simulink model "estimate_lane_center"  (R2019b)
settings: Solver=VariableStepAuto  StartTime=0.0  StopTime=10.0  RelTol=1e-3
undefined symbols (not defined in the file): PredictionHorizon, Ts
settings Model: Creator=senoa95  LastModifiedBy=senoa95

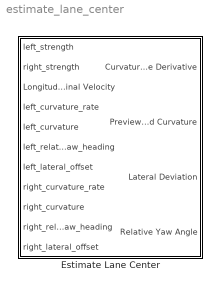
== system estimate_lane_center ==
  Estimate Lane Center : Subsystem  TreatAsAtomicUnit=on  VariantControl=v2
      settings: RTWFileNameOpts=Use function name

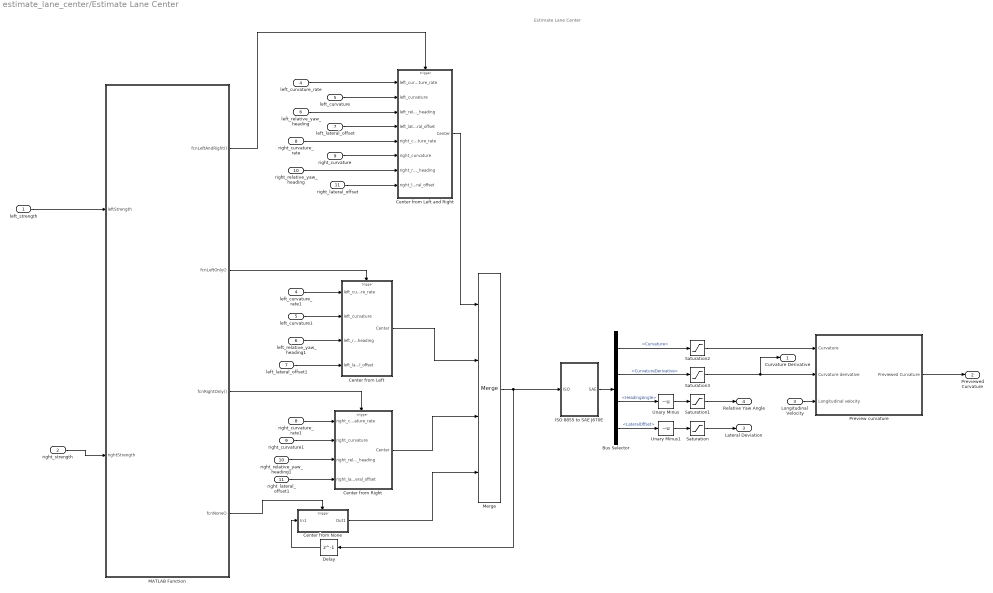
== system estimate_lane_center/Estimate Lane Center ==
  note: Estimate Lane Center
  left_strength : Inport
  right_strength : Inport  Port=2
  Longitudinal Velocity : Inport  Port=3
  left_curvature_rate : Inport  Port=4
  left_curvature : Inport  Port=5
  left_relative_yaw_heading : Inport  Port=6
  left_lateral_offset : Inport  Port=7
  right_curvature_rate : Inport  Port=8
  right_curvature : Inport  Port=9
  right_relative_yaw_heading : Inport  Port=10
  right_lateral_offset : Inport  Port=11
  Bus Selector : BusSelector  OutputSignals=Curvature,CurvatureDerivative,HeadingAngle,LateralOffset
  Center from Left : Subsystem  TreatAsAtomicUnit=on
  Center from Left and Right : Subsystem  TreatAsAtomicUnit=on
  Center from None : Subsystem  TreatAsAtomicUnit=on
  Center from Right : Subsystem  TreatAsAtomicUnit=on
  Delay : Delay  DelayLength=1
  ISO 8855 to SAE J670E : Subsystem
  MATLAB Function : MATLAB Function  TreatAsAtomicUnit=on
  Merge : Merge  Inputs=4
  Preview curvature : Subsystem
  Saturation : Saturate
  Saturation1 : Saturate  UpperLimit=0.6  LowerLimit=-0.6
  Saturation2 : Saturate  UpperLimit=0.15  LowerLimit=-0.15
  Saturation3 : Saturate  UpperLimit=0.06  LowerLimit=-0.06
  Unary Minus : UnaryMinus
  Unary Minus1 : UnaryMinus
  left_curvature1 : InportShadow  Port=5
  left_curvature_rate1 : InportShadow  Port=4
  left_lateral_offset1 : InportShadow  Port=7
  left_relative_yaw_heading1 : InportShadow  Port=6
  right_curvature1 : InportShadow  Port=9
  right_curvature_rate1 : InportShadow  Port=8
  right_lateral_offset1 : InportShadow  Port=11
  right_relative_yaw_heading1 : InportShadow  Port=10
  Curvature Derivative : Outport
  Previewed Curvature : Outport  Port=2  VectorParamsAs1DForOutWhenUnconnected=off
  Lateral Deviation : Outport  Port=3  VectorParamsAs1DForOutWhenUnconnected=off
  Relative Yaw Angle : Outport  Port=4  VectorParamsAs1DForOutWhenUnconnected=off
  wires:
  Center from Right/1(Center) -> Merge/3
  MATLAB Function/2(fcnLeftOnly()) -> Center from Left/Trigger
  Center from None/1(Out1) -> Merge/4
  MATLAB Function/1(fcnLeftAndRight()) -> Center from Left and Right/Trigger
  Delay/1 -> Center from None/1(In1)
  Center from Left and Right/1(Center) -> Merge/1
  MATLAB Function/3(fcnRightOnly()) -> Center from Right/Trigger
  MATLAB Function/4(fcnNone()) -> Center from None/Trigger
  Center from Left/1(Center) -> Merge/2
  Merge/1 -> ISO 8855 to SAE J670E/1(ISO), Delay/1
  Saturation3/1 -> Curvature Derivative/1, Preview curvature/2(Curvature derivative)
  Saturation2/1 -> Preview curvature/1(Curvature)
  Saturation1/1 -> Relative Yaw Angle/1
  Saturation/1 -> Lateral Deviation/1
  Unary Minus/1 -> Saturation1/1
  Preview curvature/1(Previewed Curvature) -> Previewed Curvature/1
  Longitudinal Velocity/1 -> Preview curvature/3(Longitudinal velocity)
  Bus Selector/2 -> Saturation3/1  "<CurvatureDerivative>"
  Bus Selector/1 -> Saturation2/1  "<Curvature>"
  Unary Minus1/1 -> Saturation/1
  Bus Selector/4 -> Unary Minus1/1  "<LateralOffset>"
  Bus Selector/3 -> Unary Minus/1  "<HeadingAngle>"
  ISO 8855 to SAE J670E/1(SAE) -> Bus Selector/1
  left_strength/1 -> MATLAB Function/1(leftStrength)
  right_strength/1 -> MATLAB Function/2(rightStrength)
  left_curvature_rate/1 -> Center from Left and Right/1(left_curvature_rate)
  right_relative_yaw_heading/1 -> Center from Left and Right/7(right_relative_yaw_heading)
  right_lateral_offset/1 -> Center from Left and Right/8(right_lateral_offset)
  left_lateral_offset/1 -> Center from Left and Right/4(left_lateral_offset)
  left_curvature/1 -> Center from Left and Right/2(left_curvature)
  left_relative_yaw_heading/1 -> Center from Left and Right/3(left_relative_yaw_heading)
  right_curvature_rate/1 -> Center from Left and Right/5(right_curvature_rate)
  right_curvature/1 -> Center from Left and Right/6(right_curvature)
  left_curvature_rate1/1 -> Center from Left/1(left_curvature_rate)
  left_curvature1/1 -> Center from Left/2(left_curvature)
  left_relative_yaw_heading1/1 -> Center from Left/3(left_relative_yaw_heading)
  left_lateral_offset1/1 -> Center from Left/4(left_lateral_offset)
  right_curvature_rate1/1 -> Center from Right/1(right_curvature_rate)
  right_curvature1/1 -> Center from Right/2(right_curvature)
  right_relative_yaw_heading1/1 -> Center from Right/3(right_relative_yaw_heading)
  right_lateral_offset1/1 -> Center from Right/4(right_lateral_offset)

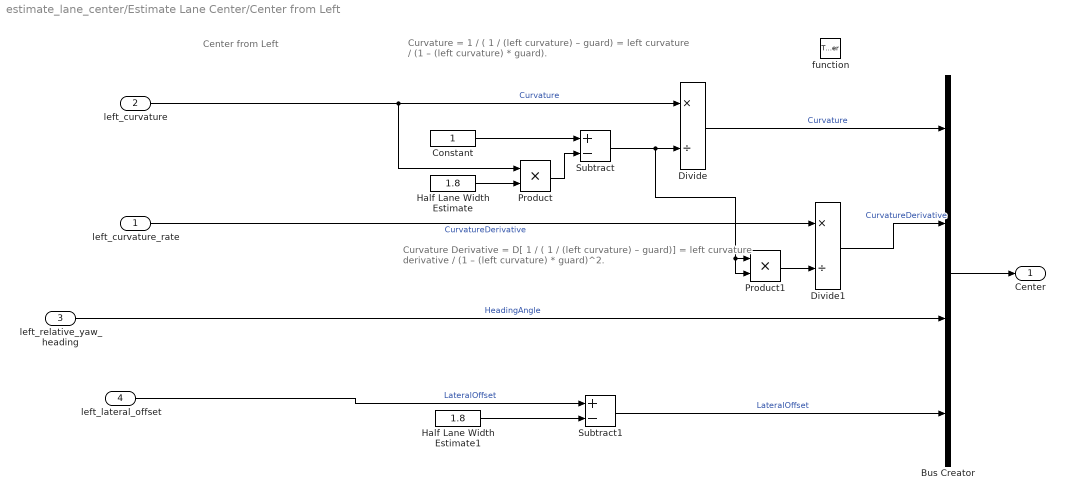
== system estimate_lane_center/Estimate Lane Center/Center from Left ==
  note: Curvature Derivative
      | = D[ 1 / ( 1 / (left curvature) – guard)]
      | = left curvature derivative / (1 – (left curvature) * guard)^2.
  note: Center from Left
  note: Curvature
      | = 1 / ( 1 / (left curvature) – guard)
      | = left curvature / (1 – (left curvature) * guard).
  left_curvature_rate : Inport
  left_curvature : Inport  Port=2
  left_relative_yaw_heading : Inport  Port=3
  left_lateral_offset : Inport  Port=4
  function : TriggerPort  TriggerType=function-call  VariantControl=Variant
  Bus Creator : BusCreator  Inputs=4
  Constant : Constant  OutDataTypeStr=Inherit: Inherit via back propagation
  Divide : Product  Inputs=*/
  Divide1 : Product  Inputs=*/
  Half Lane Width Estimate : Constant  Value=1.8  OutDataTypeStr=Inherit: Inherit via back propagation
  Half Lane Width Estimate1 : Constant  Value=1.8  OutDataTypeStr=Inherit: Inherit via back propagation
  Product : Product
  Product1 : Product
  Subtract : Sum  Inputs=+-
  Subtract1 : Sum  Inputs=+-
  Center : Outport  VectorParamsAs1DForOutWhenUnconnected=off
  wires:
  Product/1 -> Subtract/2
  Half Lane Width Estimate1/1 -> Subtract1/2
  left_lateral_offset/1 -> Subtract1/1  "LateralOffset"
  Product1/1 -> Divide1/2
  left_curvature_rate/1 -> Divide1/1  "CurvatureDerivative"
  Constant/1 -> Subtract/1
  Half Lane Width Estimate/1 -> Product/2
  Subtract/1 -> Divide/2, Product1/1, Product1/2
  left_curvature/1 -> Divide/1, Product/1  "Curvature"
  Subtract1/1 -> Bus Creator/4  "LateralOffset"
  left_relative_yaw_heading/1 -> Bus Creator/3  "HeadingAngle"
  Divide/1 -> Bus Creator/1  "Curvature"
  Divide1/1 -> Bus Creator/2  "CurvatureDerivative"
  Bus Creator/1 -> Center/1

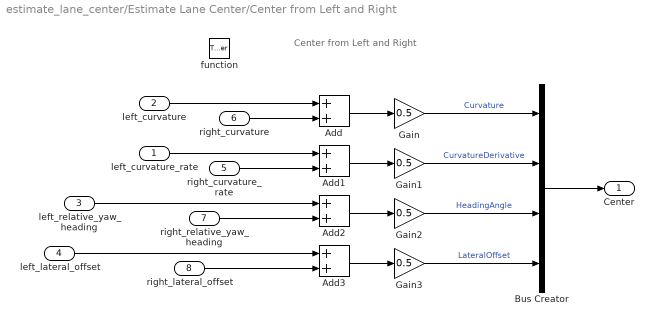
== system estimate_lane_center/Estimate Lane Center/Center from Left and Right ==
  note: Center from Left and Right
  left_curvature_rate : Inport
  left_curvature : Inport  Port=2
  left_relative_yaw_heading : Inport  Port=3
  left_lateral_offset : Inport  Port=4
  right_curvature_rate : Inport  Port=5
  right_curvature : Inport  Port=6
  right_relative_yaw_heading : Inport  Port=7
  right_lateral_offset : Inport  Port=8
  function : TriggerPort  TriggerType=function-call  VariantControl=Variant
  Add{,1..3} (4 alike) : Sum
  Bus Creator : BusCreator  Inputs=4
  Gain{,1..3} (4 alike) : Gain  Gain=0.5
  Center : Outport  VectorParamsAs1DForOutWhenUnconnected=off
  wires:
  left_lateral_offset/1 -> Add3/1
  right_lateral_offset/1 -> Add3/2
  right_relative_yaw_heading/1 -> Add2/2
  left_relative_yaw_heading/1 -> Add2/1
  right_curvature_rate/1 -> Add1/2
  left_curvature_rate/1 -> Add1/1
  left_curvature/1 -> Add/1
  Bus Creator/1 -> Center/1
  Gain3/1 -> Bus Creator/4  "LateralOffset"
  Add3/1 -> Gain3/1
  Gain2/1 -> Bus Creator/3  "HeadingAngle"
  Add2/1 -> Gain2/1
  Gain1/1 -> Bus Creator/2  "CurvatureDerivative"
  Add1/1 -> Gain1/1
  Gain/1 -> Bus Creator/1  "Curvature"
  Add/1 -> Gain/1
  right_curvature/1 -> Add/2

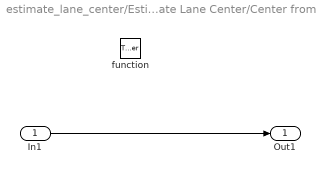
== system estimate_lane_center/Estimate Lane Center/Center from None ==
  In1 : Inport
  function : TriggerPort  TriggerType=function-call  VariantControl=Variant
  Out1 : Outport  VectorParamsAs1DForOutWhenUnconnected=off
  wires:
  In1/1 -> Out1/1

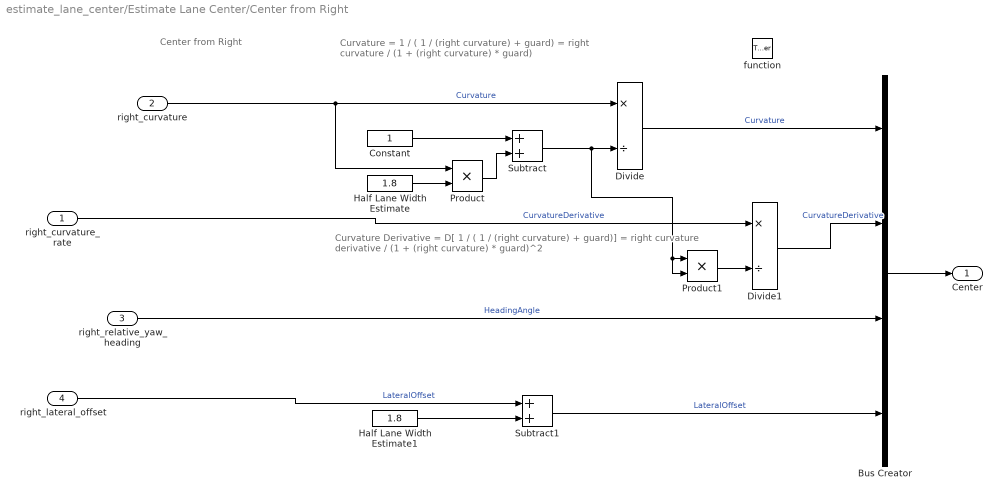
== system estimate_lane_center/Estimate Lane Center/Center from Right ==
  note: Curvature Derivative
      | = D[ 1 / ( 1 / (right curvature) + guard)]
      | = right curvature derivative / (1 + (right curvature) * guard)^2
  note: Curvature
      | = 1 / ( 1 / (right curvature) + guard)
      | = right curvature / (1 + (right curvature) * guard)
  note: Center from Right
  right_curvature_rate : Inport
  right_curvature : Inport  Port=2
  right_relative_yaw_heading : Inport  Port=3
  right_lateral_offset : Inport  Port=4
  function : TriggerPort  TriggerType=function-call  VariantControl=Variant
  Bus Creator : BusCreator  Inputs=4
  Constant : Constant  OutDataTypeStr=Inherit: Inherit via back propagation
  Divide : Product  Inputs=*/
  Divide1 : Product  Inputs=*/
  Half Lane Width Estimate : Constant  Value=1.8  OutDataTypeStr=Inherit: Inherit via back propagation
  Half Lane Width Estimate1 : Constant  Value=1.8  OutDataTypeStr=Inherit: Inherit via back propagation
  Product : Product
  Product1 : Product
  Subtract : Sum
  Subtract1 : Sum
  Center : Outport  VectorParamsAs1DForOutWhenUnconnected=off
  wires:
  Half Lane Width Estimate/1 -> Product/2
  Product/1 -> Subtract/2
  Constant/1 -> Subtract/1
  Subtract/1 -> Divide/2, Product1/1, Product1/2
  right_curvature/1 -> Divide/1, Product/1  "Curvature"
  Bus Creator/1 -> Center/1
  Subtract1/1 -> Bus Creator/4  "LateralOffset"
  Divide/1 -> Bus Creator/1  "Curvature"
  right_lateral_offset/1 -> Subtract1/1  "LateralOffset"
  Half Lane Width Estimate1/1 -> Subtract1/2
  right_relative_yaw_heading/1 -> Bus Creator/3  "HeadingAngle"
  Product1/1 -> Divide1/2
  Divide1/1 -> Bus Creator/2  "CurvatureDerivative"
  right_curvature_rate/1 -> Divide1/1  "CurvatureDerivative"

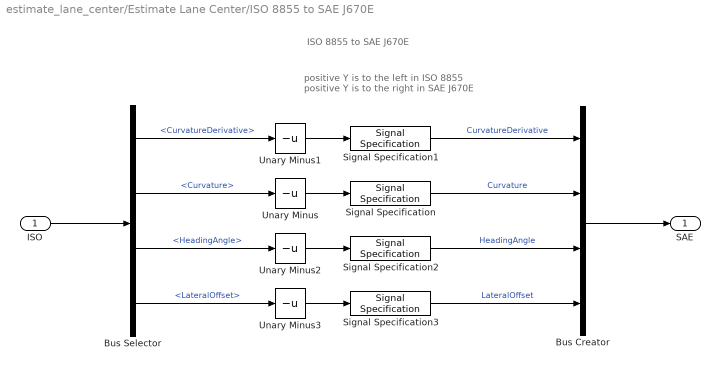
== system estimate_lane_center/Estimate Lane Center/ISO 8855 to SAE J670E ==
  note: positive Y is to the left in ISO 8855
      | positive Y is to the right in SAE J670E
  note: ISO 8855 to SAE J670E
  ISO : Inport
  Bus Creator : BusCreator  Inputs=4
  Bus Selector : BusSelector  OutputSignals=CurvatureDerivative,Curvature,HeadingAngle,LateralOffset
  Signal Specification : SignalSpecification  Unit=1/m^2
  Signal Specification1 : SignalSpecification  Unit=1/m
  Signal Specification2 : SignalSpecification  Unit=rad
  Signal Specification3 : SignalSpecification  Unit=m
  Unary Minus{,1..3} (4 alike) : UnaryMinus
  SAE : Outport  VectorParamsAs1DForOutWhenUnconnected=off
  wires:
  ISO/1 -> Bus Selector/1
  Bus Selector/2 -> Unary Minus/1  "<Curvature>"
  Bus Selector/1 -> Unary Minus1/1  "<CurvatureDerivative>"
  Bus Selector/3 -> Unary Minus2/1  "<HeadingAngle>"
  Bus Selector/4 -> Unary Minus3/1  "<LateralOffset>"
  Bus Creator/1 -> SAE/1
  Signal Specification/1 -> Bus Creator/2  "Curvature"
  Unary Minus1/1 -> Signal Specification1/1
  Unary Minus2/1 -> Signal Specification2/1
  Unary Minus3/1 -> Signal Specification3/1
  Unary Minus/1 -> Signal Specification/1
  Signal Specification1/1 -> Bus Creator/1  "CurvatureDerivative"
  Signal Specification2/1 -> Bus Creator/3  "HeadingAngle"
  Signal Specification3/1 -> Bus Creator/4  "LateralOffset"

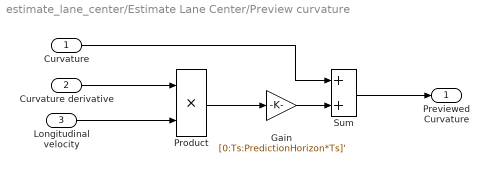
== system estimate_lane_center/Estimate Lane Center/Preview curvature ==
  Curvature : Inport
  Curvature derivative : Inport  Port=2
  Longitudinal velocity : Inport  Port=3
  Gain : Gain  Gain=[0:Ts:PredictionHorizon*Ts]'
  Product : Product
  Sum : Sum
  Previewed Curvature : Outport  VectorParamsAs1DForOutWhenUnconnected=off
  wires:
  Sum/1 -> Previewed Curvature/1
  Curvature/1 -> Sum/1
  Gain/1 -> Sum/2
  Product/1 -> Gain/1
  Longitudinal velocity/1 -> Product/2
  Curvature derivative/1 -> Product/1

== matlab function estimate_lane_center/Estimate Lane Center/MATLAB Function ==
  data: leftStrength input; rightStrength input
  events: fcnLeftAndRight output FUNCTION_CALL_EVENT; fcnLeftOnly output FUNCTION_CALL_EVENT; fcnRightOnly output FUNCTION_CALL_EVENT; fcnNone output FUNCTION_CALL_EVENT
function fcn(leftStrength,rightStrength)

% leftStrength  = lanes.Left.Strength;
% rightStrength = lanes.Right.Strength;

if (leftStrength > 0) && (rightStrength > 0)
   fcnLeftAndRight();
   
elseif leftStrength > 0
    fcnLeftOnly();
    
elseif rightStrength > 0
    fcnRightOnly();
    
else
    fcnNone();
end
